simulink model "Tanks_OP"  (R2023a)
settings: Solver=VariableStepAuto  StartTime=0.0  StopTime=10.0  RelTol=1e-3
undefined symbols (not defined in the file or in its folder): A1, A2, c1, c2, h1o, h2o
settings Model: Creator=m260477  LastModifiedBy=m260477
settings DataIOCC: Refine=10

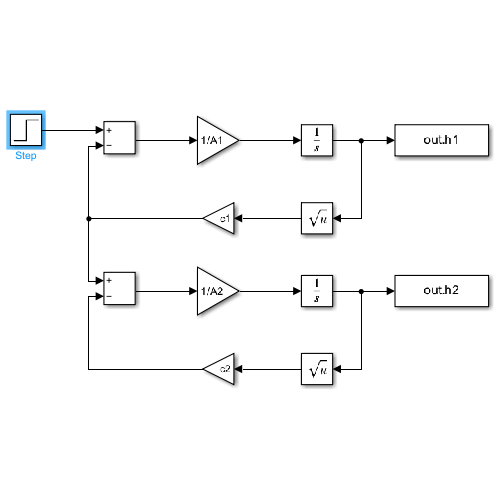
[thumbnail: Simulink's stored preview of the top-level diagram]
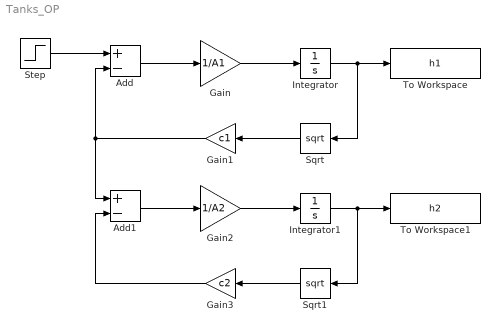
== system Tanks_OP ==
  Add : Sum  Inputs=+-
  Add1 : Sum  Inputs=+-
  Gain : Gain  Gain=1/A1
  Gain1 : Gain  Gain=c1
  Gain2 : Gain  Gain=1/A2
  Gain3 : Gain  Gain=c2
  Integrator : Integrator  InitialCondition=h1o
  Integrator1 : Integrator  InitialCondition=h2o
  Sqrt : Sqrt
  Sqrt1 : Sqrt
  Step : Step  Time=0  Before=20  After=23  SampleTime=0
  To Workspace : ToWorkspace  VariableName=h1  SaveFormat=Timeseries  SampleTime=-1
  To Workspace1 : ToWorkspace  VariableName=h2  SaveFormat=Timeseries  SampleTime=-1
  wires:
  Gain/1 -> Integrator/1
  Integrator/1 -> Sqrt/1, To Workspace/1
  Sqrt/1 -> Gain1/1
  Add/1 -> Gain/1
  Gain1/1 -> Add1/1, Add/2
  Gain3/1 -> Add1/2
  Add1/1 -> Gain2/1
  Integrator1/1 -> Sqrt1/1, To Workspace1/1
  Sqrt1/1 -> Gain3/1
  Gain2/1 -> Integrator1/1
  Step/1 -> Add/1
